simulink model "simulation_servo_agent_1219"  (R2017b)
settings: Solver=FixedStepDiscrete  StartTime=0.0  StopTime=3  FixedStep=Ts  MaxStep=1e-2  RelTol=1e-3  AbsTol=1e-3
PreLoadFcn:
  | pe_dc_motor_control_data;
values from neighbouring files (symbols this model uses):
  K = 0.00648887065107    [best_params.mat]    (also in parameter_twiddle_fast_kr.m = params(1))
  R = 5.66592438851    [best_params.mat]    (also in parameter_twiddle_fast_kr.m = params(2))
  req_speed = i    [V_P_T_simulation.m]    (also in calc_err.m; calc_err_kr.m; max_torque_at_given_speed_test.m; multi_speed_simulation.m)
  req_torque = torque_list(j)    [V_P_T_simulation.m]    (also in max_torque_at_given_speed_test.m = j; multi_speed_simulation.m = 0; parameter_twiddle_fast.m = 0)
  Tout = 0.01    [best_params.mat]
  Ts = 0.001    [best_params.mat]
undefined symbols (not defined in the file or in its folder): Linear
libraries: fl_lib x21, nesl_utility x10, robotlib x6, simulink x1, powerlib_meascontrol x1, commchan3 x1, dspstat3 x1, sdl_lib x1
Description:
  | DC Motor Control
  | 
  | This example shows a cascade speed-control structure for a DC motor.
  | A PWM controlled four-quadrant Chopper is used to feed the DC motor.
  | The Control subsystem includes the outer speed-control loop, the inner
  | current-control loop, and the PWM generation. The total simulation
  | time (t) is 4 seconds. At t = 1.5 seconds, the load torque increases.
  | At t = 2.5 seconds, the reference speed is changed from 1000 rpm to
  | 2000 rpm.
  | 
  | Copyright 2016-2017 The MathWorks, Inc.
settings Model: Creator=The MathWorks, Inc.  LastModifiedBy=s158031
settings OptimizationCC: EnhancedBackFolding=on  PassReuseOutputArgsThreshold=0  MaxStackSize=64  OptimizeBlockOrder=speed  DifferentSizesBufferReuse=on
settings DebuggingCC: UnderspecifiedInitializationDetection=Classic  MergeDetectMultiDrivingBlocksExec=none  ParameterTunabilityLossMsg=error  SFUnexpectedBacktrackingDiag=warning  SFNoUnconditionalDefaultTransitionDiag=warning  SFExecutionAtInitializationDiag=none
settings HardwareCC: ProdBitPerPointer=32  ProdBitPerSizeT=32  ProdBitPerPtrDiffT=32  ProdLargestAtomicFloat=None  ProdIntDivRoundTo=Undefined  ProdEndianess=Unspecified  ProdWordSize=32  ProdHWDeviceType=Generic->Unspecified (assume 32-bit Generic)
settings SFSimCC: MATLABDynamicMemAlloc=off
settings RTWCC: SystemTargetFile=ert.tlc  HardwareBoard=Robot Operating System (ROS)  TemplateMakefile=ert_default_tmf  GenerateReport=on  Toolchain=Catkin  LaunchReport=on  TargetLang=C++
settings CodeAppCC: ForceParamTrailComments=on  OperatorAnnotations=on
settings ERTTargetCC: ERTCustomFileBanners=off  SupportContinuousTime=on  SupportNonInlinedSFcns=on  RemoveResetFunc=off  ModelStepFunctionPrototypeControlCompliant=off
settings ConfigComp: CovMetricSettings=dw  CovHtmlReporting=on  CovSaveCumulativeToWorkspaceVar=on  CovSaveSingleToWorkspaceVar=on  CovExternalEMLEnable=off
settings SimscapeCC: SimscapeLogName=simlog_pe_dc_motor_control  SimscapeLogLimitData=off

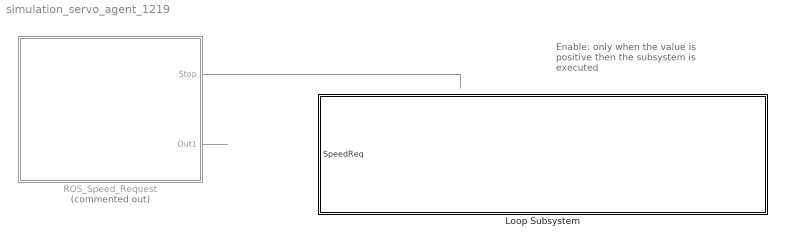
== system simulation_servo_agent_1219 ==
  note: Enable: only when the value is positive then the subsystem is executed
  Loop Subsystem : Subsystem
  ROS_Speed_Request : Subsystem  Commented=on
  wires:
  ROS_Speed_Request/2(Out1) -> ?
  ROS_Speed_Request/1(Stop) -> ?

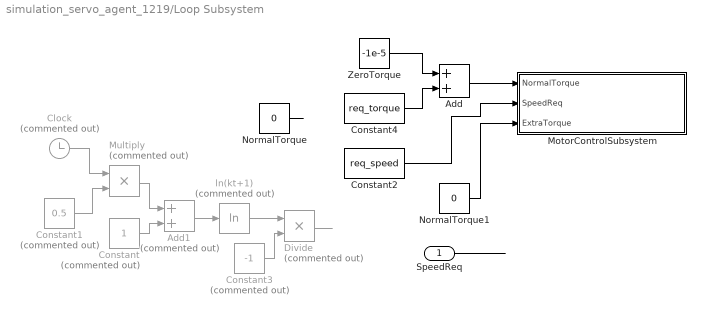
== system simulation_servo_agent_1219/Loop Subsystem ==
  "SpeedReq " : Inport
  Add : Sum
  Add1 : Sum  Commented=on
  Clock : Clock  Commented=on
  Constant : Constant  Commented=on
  Constant1 : Constant  Commented=on  Value=0.5  SampleTime=-1
  Constant2 : Constant  Value=req_speed
  Constant3 : Constant  Commented=on  Value=-1
  Constant4 : Constant  Value=req_torque
  Divide : Product  Commented=on  Inputs=**
  MotorControlSubsystem : Subsystem  TreatAsAtomicUnit=on
  Multiply : Product  Commented=on  Inputs=**
  NormalTorque : Constant  Value=0
  NormalTorque1 : Constant  Value=0
  ZeroTorque : Constant  Value=-1e-5
  ln(kt+1) : Math  Commented=on  Operator=log  SaturateOnIntegerOverflow=on
  wires:
  "SpeedReq "/1 -> ?
  Constant2/1 -> MotorControlSubsystem/2(SpeedReq)
  NormalTorque/1 -> ?
  Clock/1 -> Multiply/1
  Constant/1 -> Add1/2
  Add1/1 -> ln(kt+1)/1
  Constant1/1 -> Multiply/2
  Multiply/1 -> Add1/1
  NormalTorque1/1 -> MotorControlSubsystem/3(ExtraTorque)
  ln(kt+1)/1 -> Divide/1
  Constant3/1 -> Divide/2
  Divide/1 -> ?
  Constant4/1 -> Add/2
  ZeroTorque/1 -> Add/1
  Add/1 -> MotorControlSubsystem/1(NormalTorque)

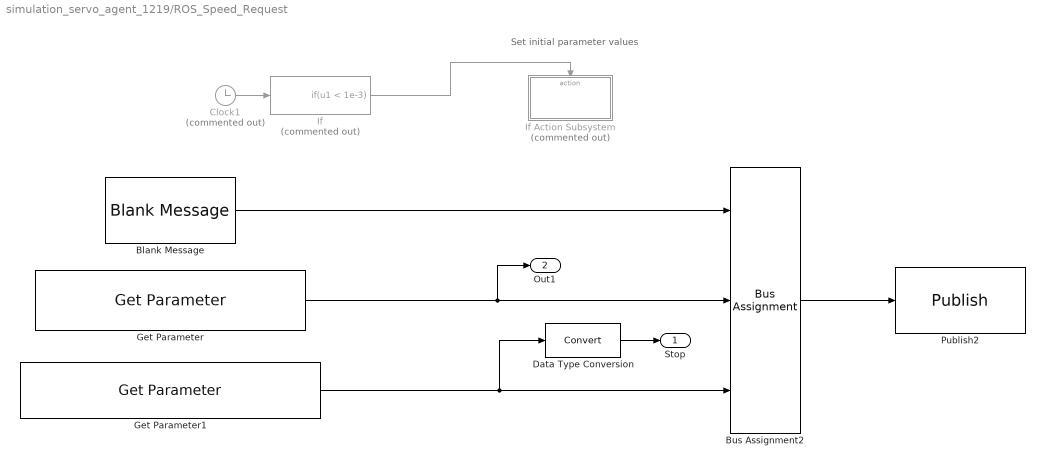
== system simulation_servo_agent_1219/ROS_Speed_Request ==
  note: Set initial parameter values
  Blank Message : robotlib/Blank Message  SourceLibraryInfo=This block requires Robotics System Toolbox  messageType=geometry_msgs/Twist  SampleTime=inf
      settings: SourceProductBaseCode=RO
  Bus Assignment2 : BusAssignment  AssignedSignals=Linear.X,Linear.Y
  Clock1 : Clock  Commented=on
  Data Type Conversion : DataTypeConversion
  Get Parameter : robotlib/Get Parameter  SourceLibraryInfo=This block requires Robotics System Toolbox  ParameterSource=Select from ROS network  ParameterName=/simulation_servo_agent/update_velocity/speed  ParameterType=double  ParameterMaxArrayLength=16  ParameterInitialValue=0.0  SampleTime=-1  ShowErrorCodeOutput=off  ModelName=simulation_servo_agent_928  BlockId=ParamGet_simulation_servo_agent_928_3318
      settings: SourceProductName=Robotics System Toolbox  SourceProductBaseCode=RO
  Get Parameter1 : robotlib/Get Parameter  SourceLibraryInfo=This block requires Robotics System Toolbox  ParameterSource=Select from ROS network  ParameterName=/simulation_servo_agent/update_velocity/isEnabled  ParameterType=double  ParameterMaxArrayLength=16  ParameterInitialValue=0.0  SampleTime=-1  ShowErrorCodeOutput=off  ModelName=simulation_servo_agent_928  BlockId=ParamGet_simulation_servo_agent_928_3398
      settings: SourceProductName=Robotics System Toolbox  SourceProductBaseCode=RO
  If : If  Commented=on  IfExpression=u1 < 1e-3  ShowElse=off
  If Action Subsystem : Subsystem  Commented=on  TreatAsAtomicUnit=on
  Publish2 : robotlib/Publish  SourceLibraryInfo=This block requires Robotics System Toolbox  topicSource=Specify your own  topic=/my_speed  messageType=geometry_msgs/Twist  messageQueueLength=105
      settings: SourceProductBaseCode=RO
  Stop : Outport
  Out1 : Outport  Port=2
  wires:
  Get Parameter/1 -> Out1/1, Bus Assignment2/2
  Bus Assignment2/1 -> Publish2/1
  Blank Message/1 -> Bus Assignment2/1
  Get Parameter1/1 -> Data Type Conversion/1, Bus Assignment2/3
  Data Type Conversion/1 -> Stop/1
  Clock1/1 -> If/1
  If/1 -> If Action Subsystem/Action

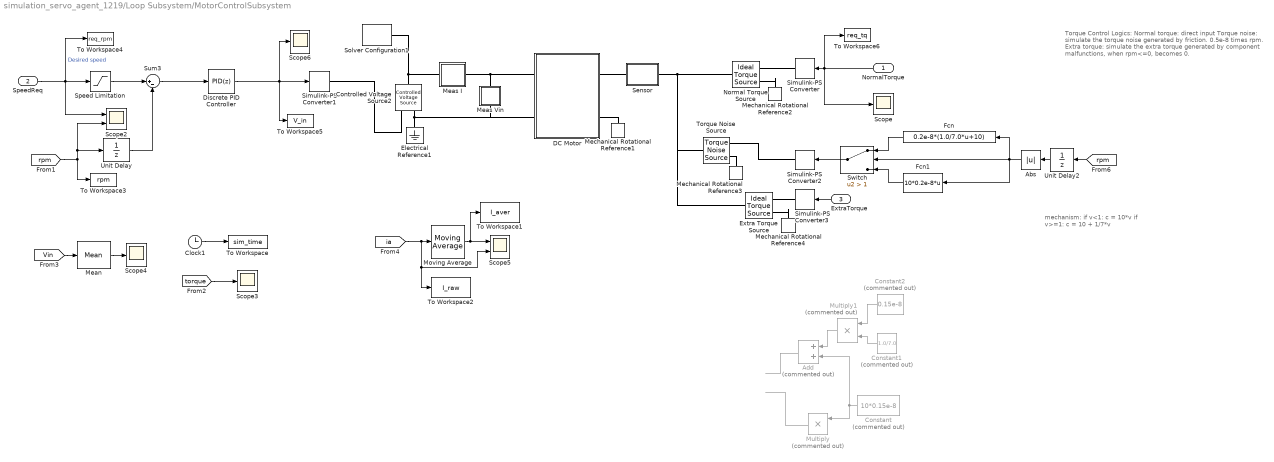
== system simulation_servo_agent_1219/Loop Subsystem/MotorControlSubsystem ==
  note: mechanism:
      | if v<1: c = 10*v
      | if v>=1: c = 10 + 1/7*v
  note: Torque Control Logics:
      | Normal torque: direct input
      | Torque noise: simulate the torque noise generated by friction. 0.5e-8 times rpm.
      | Extra torque: simulate the extra torque generated by component malfunctions, when rpm<=0, becomes 0.
  NormalTorque : Inport
  SpeedReq : Inport  Port=2
  ExtraTorque : Inport  Port=3
  Abs : Abs
  Add : Sum  Commented=on
  Clock1 : Clock
  Constant : Constant  Commented=on  Value=10*0.15e-8
  Constant1 : Constant  Commented=on  Value=1.0/7.0
  Constant2 : Constant  Commented=on  Value=0.15e-8
  Controlled Voltage Source2 : fl_lib/Electrical/Electrical Sources/Controlled Voltage Source
  DC Motor : Subsystem
  Discrete PID Controller : simulink/Continuous/PID Controller  Controller=PID  TimeDomain=Discrete-time  SampleTime=-1  IntegratorMethod=Forward Euler  FilterMethod=Forward Euler  Form=Parallel  UseFilter=on  ControllerParametersSource=internal  P=0.12  I=1.5  D=0.007  N=55  InitialConditionSource=internal  InitialConditionForIntegrator=0  InitialConditionForFilter=0  ExternalReset=none  LimitOutput=on  UpperSaturationLimit=11.1  LowerSaturationLimit=-11.1  LinearizeAsGain=off  AntiWindupMode=none  Kb=1  TrackingMode=off  Kt=1  PParamMin=[]  PParamMax=[]  IParamMin=[]  IParamMax=[]  DParamMin=[]  DParamMax=[]  NParamMin=[]  NParamMax=[]  KbParamMin=[]  KbParamMax=[]  KtParamMin=[]  KtParamMax=[]  POutMin=[]  POutMax=[]  IOutMin=[]  IOutMax=[]  DOutMin=[]  DOutMax=[]  NOutMin=[]  NOutMax=[]  KbOutMin=[]  KbOutMax=[]  KtOutMin=[]  KtOutMax=[]  IntegratorOutMin=[]  IntegratorOutMax=[]  FilterOutMin=[]  FilterOutMax=[]  SumOutMin=[]  SumOutMax=[]  SumI1OutMin=[]  SumI1OutMax=[]  SumI2OutMin=[]  SumI2OutMax=[]  SumI3OutMin=[]  SumI3OutMax=[]  SumDOutMin=[]  SumDOutMax=[]  SaturationOutMin=[]  SaturationOutMax=[]  IntegratorContinuousStateAttributes=''  IntegratorStateMustResolveToSignalObject=off  IntegratorRTWStateStorageClass=Auto  FilterContinuousStateAttributes=''  FilterStateMustResolveToSignalObject=off  FilterRTWStateStorageClass=Auto  DifferentiatorICPrevScaledInput=0  DifferentiatorOutMin=[]  DifferentiatorOutMax=[]  InitialConditionSetting=State (most efficient)  FilterDiffOutCoefMin=[]  FilterDiffOutCoefMax=[]  SumDenOutMin=[]  SumDenOutMax=[]  SumNumOutMin=[]  SumNumOutMax=[]  ReciprocalOutMin=[]  ReciprocalOutMax=[]  DivideOutMin=[]  DivideOutMax=[]  TunerSelectOption=Transfer Function Based (PID Tuner App)
  Electrical Reference1 : fl_lib/Electrical/Electrical Elements/Electrical Reference
      settings: SourceProductName=Foundation Library
  Extra Torque Source : fl_lib/Mechanical/Mechanical Sources/Ideal Torque Source
      settings: SourceProductName=Foundation Library
  Fcn : Fcn  Expr=0.2e-8*(1.0/7.0*u+10)
  Fcn1 : Fcn  Expr=10*0.2e-8*u
  Mean : powerlib_meascontrol/Measurements/Mean  Freq=10  Vinit=0  Ts=Ts
  Meas I : Subsystem
  Meas Vin : Subsystem
  Mechanical Rotational Reference{1..4} (4 alike) : fl_lib/Mechanical/Rotational Elements/Mechanical Rotational Reference
      settings: SourceProductName=Foundation Library
  Moving Average : dspstat3/Moving Average  Method=Sliding window  SpecifyWindowLength=on  WindowLength=1000  ForgettingFactor=0.9  SimulateUsing=Code generation
  Multiply : Product  Commented=on  Inputs=**
  Multiply1 : Product  Commented=on  Inputs=***
  Normal Torque Source : fl_lib/Mechanical/Mechanical Sources/Ideal Torque Source
      settings: SourceProductName=Foundation Library
  Scope{,3..4,6} (4 alike) : Scope
  Scope2 : Scope  NumInputPorts=2
  Scope5 : Scope  NumInputPorts=2
  Sensor : Subsystem
  Simulink-PS Converter{,1..3} (4 alike) : nesl_utility/Simulink-PS Converter  PhysicalDomain=network_engine_domain  SubClassName=ps_input  LeftPortType=input  RightPortType=output  PseudoPeriodic=off  Frequencies=[]  NoiseDistribution=none  NoiseParameters=[]  Unit=1  AffineConversion=off  FilteringAndDerivatives=provide  SimscapeFilterOrder=1  InputFilterTimeConstant=0.001  UdotUserProvided=0
  Solver Configuration1 : nesl_utility/Solver Configuration  PhysicalDomain=network_engine_domain  SubClassName=solver  LeftPortType=input  RightPortType=generic  Accelerate=off  Tones=[]  Harmonics=[]  SimulateNoise=off  Profile=off  UseLocalSampling=off  EnableSwitchedLinearOptims=on  FrequencyDomain=off  UseCCode=off  RelTol=0.001  AbsTol=1e-06  MinStep=1e-09  ToWorkspace=off  RevertToSquareIcSolve=off  NumHomotopyIterations=100  PhasorMode=off  PhasorModeNumHarmonics=1  DoDC=off  ResidualTolerance=1e-09  UseLocalSolver=on  LocalSolverChoice=NE_BACKWARD_EULER_ADVANCER  LocalSolverSampleTime=Ts  DoFixedCost=on  MaxNonlinIter=3  MaxModeIter=2  LinearAlgebra=Sparse  DelaysMemoryBudget=1024  AutomaticFiltering=on  FilteringTimeConstant=0.001
  Speed Limitation : Saturate  UpperLimit=57  LowerLimit=-57
  Sum3 : Sum  Inputs=|+-
  Switch : Switch  Criteria=u2 > Threshold  Threshold=1
  To Workspace : ToWorkspace  VariableName=sim_time  SampleTime=-1
      settings: Save2DSignal=2-D array (concatenate along first dimension)
  To Workspace1 : ToWorkspace  VariableName=I_aver  SampleTime=Tout
      settings: Save2DSignal=2-D array (concatenate along first dimension)
  To Workspace2 : ToWorkspace  VariableName=I_raw  SampleTime=Tout
  To Workspace3 : ToWorkspace  VariableName=rpm  SampleTime=Tout
      settings: Save2DSignal=2-D array (concatenate along first dimension)
  To Workspace4 : ToWorkspace  VariableName=req_rpm  SampleTime=Tout
      settings: Save2DSignal=2-D array (concatenate along first dimension)
  To Workspace5 : ToWorkspace  VariableName=V_in  SampleTime=Tout
      settings: Save2DSignal=2-D array (concatenate along first dimension)
  To Workspace6 : ToWorkspace  VariableName=req_tq  SampleTime=Tout
      settings: Save2DSignal=2-D array (concatenate along first dimension)
  Torque Noise Source : sdl_lib/Sources/Torque Noise Source  sample_time=1e-3 s  repeatability=3  user_seed=0  auto_seed=3499211588
      settings: SourceProductName=Simscape Driveline  SourceProductBaseCode=LD
  Unit Delay : UnitDelay  SampleTime=Ts
  Unit Delay2 : UnitDelay  SampleTime=Ts
  wires:
  SpeedReq/1 -> To Workspace4/1, Speed Limitation/1, Scope2/1  "Desired speed"
  NormalTorque/1 -> To Workspace6/1, Simulink-PS Converter/1, Scope/1
  [Vin] -> Mean/1
  Moving Average/1 -> To Workspace1/1, Scope5/1
  Mean/1 -> Scope4/1
  Unit Delay/1 -> Sum3/2
  Clock1/1 -> To Workspace/1
  [torque] -> Scope3/1
  Speed Limitation/1 -> Sum3/1
  Sum3/1 -> Discrete PID Controller/1
  Discrete PID Controller/1 -> To Workspace5/1, Scope6/1, Simulink-PS Converter1/1
  ExtraTorque/1 -> Simulink-PS Converter3/1
  [ia] -> To Workspace2/1, Scope5/2, Moving Average/1
  [rpm] -> Scope2/2, Unit Delay/1, To Workspace3/1
  Unit Delay2/1 -> Abs/1
  [rpm] -> Unit Delay2/1
  Switch/1 -> Simulink-PS Converter2/1
  Multiply/1 -> ?
  Add/1 -> ?
  Multiply1/1 -> Add/1
  Constant2/1 -> Multiply1/1
  Constant/1 -> Add/2, Multiply/1
  ? -> Multiply1/2, Multiply/2
  Constant1/1 -> Multiply1/3
  Fcn1/1 -> Switch/3
  Fcn/1 -> Switch/1
  Abs/1 -> Fcn1/1, Fcn/1, Switch/2
  connections:
  Meas Vin/LConn1 -- DC Motor/LConn1 -- Meas I/RConn1
  DC Motor/RConn1 -- Sensor/LConn1
  Simulink-PS Converter/RConn1 -- Normal Torque Source/RConn1
  DC Motor/RConn2 -- Mechanical Rotational Reference1/LConn1
  Mechanical Rotational Reference2/LConn1 -- Normal Torque Source/RConn2
  Electrical Reference1/LConn1 -- Controlled Voltage Source2/RConn2 -- DC Motor/LConn2 -- Meas Vin/RConn1
  Controlled Voltage Source2/LConn1 -- Solver Configuration1/RConn1 -- Meas I/LConn1
  Controlled Voltage Source2/RConn1 -- Simulink-PS Converter1/RConn1
  Normal Torque Source/LConn1 -- Torque Noise Source/RConn1 -- Extra Torque Source/LConn1 -- Sensor/RConn1
  Simulink-PS Converter3/RConn1 -- Extra Torque Source/RConn1
  Mechanical Rotational Reference4/LConn1 -- Extra Torque Source/RConn2
  Mechanical Rotational Reference3/LConn1 -- Torque Noise Source/LConn2
  Simulink-PS Converter2/RConn1 -- Torque Noise Source/LConn1

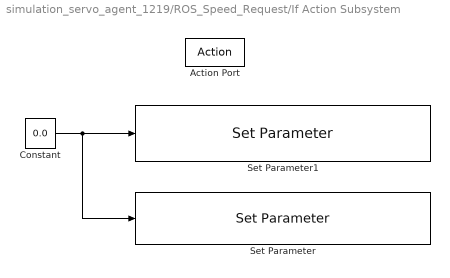
== system simulation_servo_agent_1219/ROS_Speed_Request/If Action Subsystem ==
  Action Port : ActionPort  ActionType=then
  Constant : Constant  Value=0.0
  Set Parameter : robotlib/Set Parameter  SourceLibraryInfo=This block requires Robotics System Toolbox  ParameterSource=Select from ROS network  ParameterName=/simulation_servo_agent/update_velocity/isEnabled  ParameterType=double  ModelName=simulation_servo_agent_925  BlockId=ParamSet_simulation_servo_agent_925_3446
      settings: SourceProductName=Robotics System Toolbox  SourceProductBaseCode=RO
  Set Parameter1 : robotlib/Set Parameter  SourceLibraryInfo=This block requires Robotics System Toolbox  ParameterSource=Select from ROS network  ParameterName=/simulation_servo_agent/update_velocity/speed  ParameterType=double  ModelName=simulation_servo_agent_925  BlockId=ParamSet_simulation_servo_agent_925_3447
      settings: SourceProductName=Robotics System Toolbox  SourceProductBaseCode=RO
  wires:
  Constant/1 -> Set Parameter/1, Set Parameter1/1

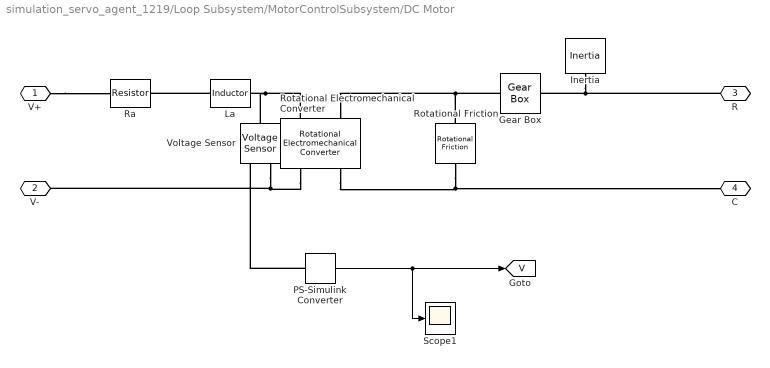
== system simulation_servo_agent_1219/Loop Subsystem/MotorControlSubsystem/DC Motor ==
  Gear Box : fl_lib/Mechanical/Mechanisms/Gear Box  ratio=258.5  t_in_specify=off  t_in_priority=None  t_in=0 N*m  t_in_nominal_specify=off  t_in_nominal_unit=N*m  t_in_nominal_value=1  t_out_specify=off  t_out_priority=None  t_out=0 N*m  t_out_nominal_specify=off  t_out_nominal_unit=N*m  t_out_nominal_value=1
  Inertia : fl_lib/Mechanical/Rotational Elements/Inertia  inertia=J kg*m^2  w_specify=off  w_priority=High  w=0 rad/s  w_nominal_specify=off  w_nominal_unit=rad/s  w_nominal_value=1  t_specify=off  t_priority=None  t=0 N*m  t_nominal_specify=off  t_nominal_unit=N*m  t_nominal_value=1
      settings: SourceProductName=Foundation Library
  La : fl_lib/Electrical/Electrical Elements/Inductor  l=L H  r=0 Ohm  g=1e-9 1/Ohm  i_specify=off  i_priority=None  i=0 A  i_nominal_specify=off  i_nominal_unit=A  i_nominal_value=1  v_specify=off  v_priority=None  v=0 V  v_nominal_specify=off  v_nominal_unit=V  v_nominal_value=1  i_L_specify=on  i_L_priority=High  i_L=0 A  i_L_nominal_specify=off  i_L_nominal_unit=A  i_L_nominal_value=1
      settings: SourceProductName=Foundation Library
  PS-Simulink Converter : nesl_utility/PS-Simulink Converter  PhysicalDomain=network_engine_domain  SubClassName=ps_output  LeftPortType=input  RightPortType=output  PseudoPeriodic=off  Frequencies=[]  Unit=1  AffineConversion=off
  Ra : fl_lib/Electrical/Electrical Elements/Resistor  R=R Ohm  i_specify=off  i_priority=None  i=0 A  i_nominal_specify=off  i_nominal_unit=A  i_nominal_value=1  v_specify=off  v_priority=None  v=0 V  v_nominal_specify=off  v_nominal_unit=V  v_nominal_value=1
      settings: SourceProductName=Foundation Library
  Rotational Electromechanical Converter : fl_lib/Electrical/Electrical Elements/Rotational Electromechanical Converter  K=K V/(rad/s)  i_specify=off  i_priority=None  i=0 A  i_nominal_specify=off  i_nominal_unit=A  i_nominal_value=1  v_specify=off  v_priority=None  v=0 V  v_nominal_specify=off  v_nominal_unit=V  v_nominal_value=1  t_specify=off  t_priority=None  t=0 N*m  t_nominal_specify=off  t_nominal_unit=N*m  t_nominal_value=1  w_specify=off  w_priority=None  w=0 rad/s  w_nominal_specify=off  w_nominal_unit=rad/s  w_nominal_value=1
      settings: SourceProductName=Foundation Library
  Rotational Friction : fl_lib/Mechanical/Rotational Elements/Rotational Friction  brkwy_trq=C N*m  brkwy_vel=1e-5 rad/s  Col_trq=C N*m  visc_coef=F N*m/(rad/s)  w_specify=off  w_priority=None  w=0 rad/s  w_nominal_specify=off  w_nominal_unit=rad/s  w_nominal_value=1  t_specify=off  t_priority=None  t=0 N*m  t_nominal_specify=off  t_nominal_unit=N*m  t_nominal_value=1
      settings: SourceProductName=Simscape
  Scope1 : Scope
  Voltage Sensor : fl_lib/Electrical/Electrical Sensors/Voltage Sensor
  V+ : PMIOPort  Port=1  Side=Left
  V- : PMIOPort  Port=2  Side=Left
  R : PMIOPort  Port=3  Side=Right
  C : PMIOPort  Port=4  Side=Right
  tag scope: V=global
  wires:
  PS-Simulink Converter/1 -> Scope1/1, [V]
  connections:
  Rotational Electromechanical Converter/RConn1 -- Voltage Sensor/RConn2 -- V-/RConn1
  V+/RConn1 -- Ra/LConn1
  Rotational Electromechanical Converter/RConn2 -- Rotational Friction/RConn1 -- C/RConn1
  Gear Box/LConn1 -- Rotational Electromechanical Converter/LConn2 -- Rotational Friction/LConn1
  R/RConn1 -- Inertia/LConn1 -- Gear Box/RConn1
  Rotational Electromechanical Converter/LConn1 -- Voltage Sensor/LConn1 -- La/RConn1
  La/LConn1 -- Ra/RConn1
  PS-Simulink Converter/LConn1 -- Voltage Sensor/RConn1

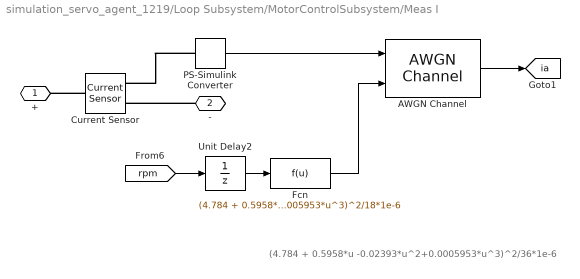
== system simulation_servo_agent_1219/Loop Subsystem/MotorControlSubsystem/Meas I ==
  note: (4.784 + 0.5958*u -0.02393*u^2+0.0005953*u^3)^2/36*1e-6
  AWGN Channel : commchan3/AWGN Channel  InputProcessing=Columns as channels (frame based)  seed=67  noiseMode=Variance from port  EbNodB=10  EsNodB=10  SNRdB=10  bitsPerSym=1  Ps=1  Tsym=1  variance=1
  Current Sensor : fl_lib/Electrical/Electrical Sensors/Current Sensor
      settings: SourceProductName=Foundation Library
  Fcn : Fcn  Expr=(4.784 + 0.5958*u -0.02393*u^2+0.0005953*u^3)^2/18*1e-6
  PS-Simulink Converter : nesl_utility/PS-Simulink Converter  PhysicalDomain=network_engine_domain  SubClassName=ps_output  LeftPortType=input  RightPortType=output  PseudoPeriodic=off  Frequencies=[]  Unit=1  AffineConversion=off
  Unit Delay2 : UnitDelay  SampleTime=Ts
  + : PMIOPort  Port=1  Side=Left
  - : PMIOPort  Port=2  Side=Right
  tag scope: ia=global
  wires:
  PS-Simulink Converter/1 -> AWGN Channel/1
  AWGN Channel/1 -> [ia]
  [rpm] -> Unit Delay2/1
  Unit Delay2/1 -> Fcn/1
  Fcn/1 -> AWGN Channel/2
  connections:
  PS-Simulink Converter/LConn1 -- Current Sensor/RConn1
  Current Sensor/LConn1 -- +/RConn1
  -/RConn1 -- Current Sensor/RConn2

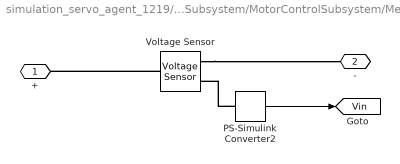
== system simulation_servo_agent_1219/Loop Subsystem/MotorControlSubsystem/Meas Vin ==
  PS-Simulink Converter2 : nesl_utility/PS-Simulink Converter  PhysicalDomain=network_engine_domain  SubClassName=ps_output  LeftPortType=input  RightPortType=output  PseudoPeriodic=off  Frequencies=[]  Unit=V  AffineConversion=off
  Voltage Sensor : fl_lib/Electrical/Electrical Sensors/Voltage Sensor
      settings: SourceProductName=Foundation Library
  + : PMIOPort  Port=1  Side=Left
  - : PMIOPort  Port=2  Side=Right
  tag scope: Vin=global
  wires:
  PS-Simulink Converter2/1 -> [Vin]
  connections:
  Voltage Sensor/LConn1 -- +/RConn1
  PS-Simulink Converter2/LConn1 -- Voltage Sensor/RConn1
  Voltage Sensor/RConn2 -- -/RConn1

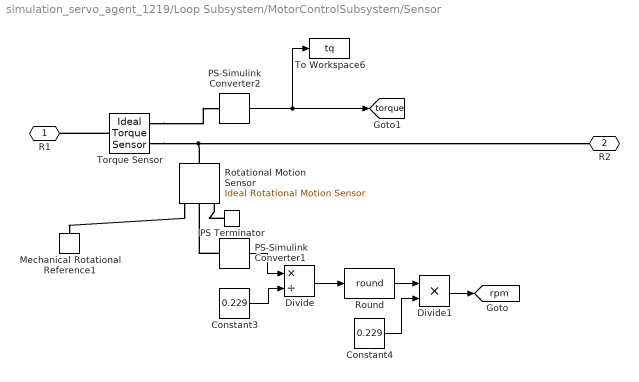
== system simulation_servo_agent_1219/Loop Subsystem/MotorControlSubsystem/Sensor ==
  Constant3 : Constant  Value=0.229
  Constant4 : Constant  Value=0.229
  Divide : Product  Inputs=*/
  Divide1 : Product  Inputs=**
  Mechanical Rotational Reference1 : fl_lib/Mechanical/Rotational Elements/Mechanical Rotational Reference
      settings: SourceProductName=Foundation Library
  PS Terminator : fl_lib/Physical Signals/Sinks/PS Terminator
      settings: SourceProductName=Foundation Library
  PS-Simulink Converter1 : nesl_utility/PS-Simulink Converter  PhysicalDomain=network_engine_domain  SubClassName=ps_output  LeftPortType=input  RightPortType=output  PseudoPeriodic=off  Frequencies=[]  Unit=rpm  AffineConversion=off
  PS-Simulink Converter2 : nesl_utility/PS-Simulink Converter  PhysicalDomain=network_engine_domain  SubClassName=ps_output  LeftPortType=input  RightPortType=output  PseudoPeriodic=off  Frequencies=[]  Unit=N*m  AffineConversion=off
  Rotational Motion Sensor : fl_lib/Mechanical/Mechanical Sensors/Ideal Rotational Motion Sensor  offset=0 rad
      settings: SourceProductName=Foundation Library
  Round : Rounding  Operator=round
  To Workspace6 : ToWorkspace  VariableName=tq  SampleTime=Tout
      settings: Save2DSignal=2-D array (concatenate along first dimension)
  Torque Sensor : fl_lib/Mechanical/Mechanical Sensors/Ideal Torque Sensor
      settings: SourceProductName=Foundation Library
  R1 : PMIOPort  Port=1  Side=Left
  R2 : PMIOPort  Port=2  Side=Right
  tag scope: rpm=global, torque=global
  wires:
  PS-Simulink Converter2/1 -> To Workspace6/1, [torque]
  Divide/1 -> Round/1
  Round/1 -> Divide1/1
  Constant3/1 -> Divide/2
  Constant4/1 -> Divide1/2
  Divide1/1 -> [rpm]
  PS-Simulink Converter1/1 -> Divide/1
  connections:
  Rotational Motion Sensor/RConn1 -- Mechanical Rotational Reference1/LConn1
  Torque Sensor/LConn1 -- R1/RConn1
  Torque Sensor/RConn2 -- PS-Simulink Converter2/LConn1
  PS-Simulink Converter1/LConn1 -- Rotational Motion Sensor/RConn2
  PS Terminator/LConn1 -- Rotational Motion Sensor/RConn3
  Torque Sensor/RConn1 -- R2/RConn1 -- Rotational Motion Sensor/LConn1
